simulink model "JXvoice"  (Simulink 7.7)
settings: Solver=ode45  StartTime=0.0  StopTime=10.0  RelTol=1e-3
undefined symbols (not defined in the file or in its folder): Fs, get, sided, Two
libraries: simulink x12, dspsrcs4 x2, dspmathops x1, dsparch4 x1, dspstat3 x1, dspsnks4 x1, dspsigops x1
settings Model: Creator=Jx  LastModifiedBy=Jx

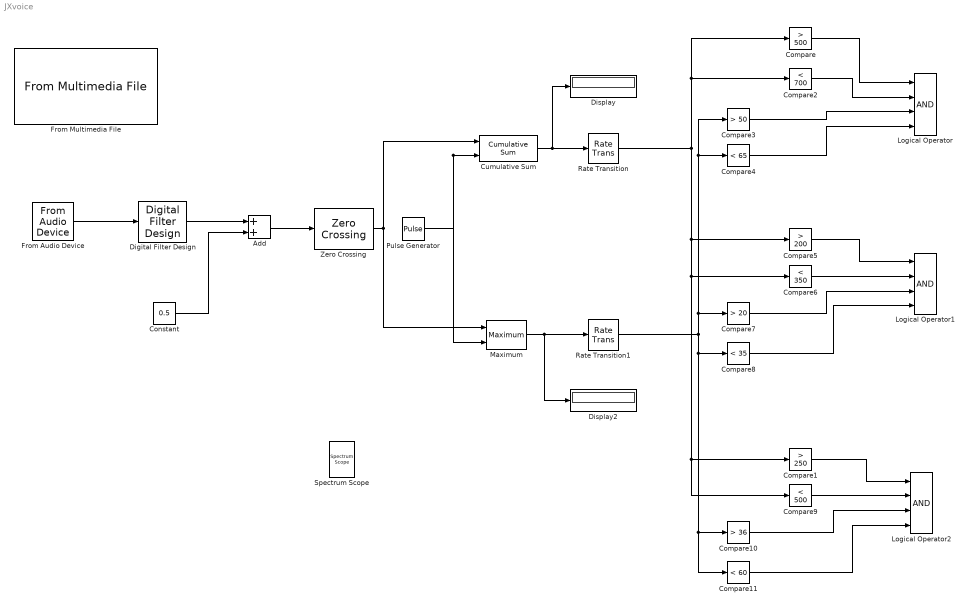
== system JXvoice ==
  Add : Sum
  Compare : simulink/Logic and Bit Operations/Compare To Constant  SystemSampleTime=-1  relop=>  const=500  LogicOutDataTypeMode=uint8
  Compare1 : simulink/Logic and Bit Operations/Compare To Constant  SystemSampleTime=-1  relop=>  const=250  LogicOutDataTypeMode=uint8
  Compare10 : simulink/Logic and Bit Operations/Compare To Constant  SystemSampleTime=-1  relop=>  const=36  LogicOutDataTypeMode=uint8
  Compare11 : simulink/Logic and Bit Operations/Compare To Constant  SystemSampleTime=-1  relop=<  const=60  LogicOutDataTypeMode=uint8
  Compare2 : simulink/Logic and Bit Operations/Compare To Constant  SystemSampleTime=-1  relop=<  const=700  LogicOutDataTypeMode=uint8
  Compare3 : simulink/Logic and Bit Operations/Compare To Constant  SystemSampleTime=-1  relop=>  const=50  LogicOutDataTypeMode=uint8
  Compare4 : simulink/Logic and Bit Operations/Compare To Constant  SystemSampleTime=-1  relop=<  const=65  LogicOutDataTypeMode=uint8
  Compare5 : simulink/Logic and Bit Operations/Compare To Constant  SystemSampleTime=-1  relop=>  const=200  LogicOutDataTypeMode=uint8
  Compare6 : simulink/Logic and Bit Operations/Compare To Constant  SystemSampleTime=-1  relop=<  const=350  LogicOutDataTypeMode=uint8
  Compare7 : simulink/Logic and Bit Operations/Compare To Constant  SystemSampleTime=-1  relop=>  const=20  LogicOutDataTypeMode=uint8
  Compare8 : simulink/Logic and Bit Operations/Compare To Constant  SystemSampleTime=-1  relop=<  const=35  LogicOutDataTypeMode=uint8
  Compare9 : simulink/Logic and Bit Operations/Compare To Constant  SystemSampleTime=-1  relop=<  const=500  LogicOutDataTypeMode=uint8
  Constant : Constant  Value=0.5
  Cumulative Sum : dspmathops/Cumulative Sum  dim=Channels (running sum)  InputProcessing=Columns as channels (frame based)  reset_popup=Either edge  outputDataTypeStr=Inherit: Same as accumulator  outputLastDataTypeStr=Inherit: Same as accumulator  outputMin=[]  outputMax=[]  roundingMode=Floor  overflowMode=off
  Digital Filter Design : dsparch4/Digital Filter Design  SystemSampleTime=-1  mwdsp_browser_bugfix_var=off
  Display : Display
  Display2 : Display
  From Audio Device : dspsrcs4/From Audio Device  deviceName=Default  numChannels=1  sampleRate=8000  deviceDatatype=24-bit integer  autoBufferSize=on  bufferSize=4096  queueDuration=1.0  frameSize=256  outputDatatype=single
  From Multimedia File : dspsrcs4/From Multimedia File  inputFilename=speech_dft.avi  loop=on  numPlays=inf  outputStreams=Audio only  videoDataType=single  audioDataType=int16  inheritSampleTime=on  userDefinedSampleTime=1/31.25  noAudioOutput=off  isIntensityVideo=off  fourcc=RGB  colorVideoFormat=Separate color signals  outputEOF=off  dataOrg=Column-major  audioFrameSize=5632  computeAudioFrameSize=off
  Logical Operator : Logic  Inputs=4  AllPortsSameDT=off  OutDataTypeStr=boolean
  Logical Operator1 : Logic  Inputs=4  AllPortsSameDT=off  OutDataTypeStr=boolean
  Logical Operator2 : Logic  Inputs=4  AllPortsSameDT=off  OutDataTypeStr=boolean
  Maximum : dspstat3/Maximum  fcn=Running  reset=Either edge  InputProcessing=Columns as channels (frame based)  indexBase=One  operateOver=Each column  Dimension=1  colComp=on  operation=maximum  roiEnable=off  roiType=Rectangles  roiPortion=Entire ROI  roiOutput=Individual statistics for each ROI  roiFlag=off  accumDataTypeStr=Inherit: Same as product output  accumLastDataTypeStr=Inherit: Same as product output  roundingMode=Floor  overflowMode=off
  Pulse Generator : DiscretePulseGenerator  SampleTime=1/31.25
  Rate Transition : RateTransition
  Rate Transition1 : RateTransition
  Spectrum Scope : dspsnks4/Spectrum Scope  SystemSampleTime=-1  ScopeProperties=on  Domain=Frequency  HorizSpan=1  UseBuffer=off  BufferSize=128  Overlap=0  TreatMby1Signals=One channel  inpFftLenInherit=off  FFTlength=128  numAvg=2  DisplayProperties=off  AxisGrid=on  Memory=off  FrameNumber=on  AxisLegend=off  AxisZoom=off  OpenScopeAtSimStart=on  OpenScopeImmediately=off  FigPos=get(0,'defaultfigureposition')  AxisProperties=off  XUnits=Hertz  XRange=Two-sided ((-Fs/2...Fs/2])  XDisplay=0  InheritXIncr=on  XIncr=1.0  XLabel=Samples  XLimit=Auto  YUnits=dBW/Hertz  XMax=1  XMin=0  YLabel=Magnitude-squared, dB  LineProperties=off  wintypeSpecScope=Hann  RsSpecScope=50  betaSpecScope=5  winsampSpecScope=Periodic  XAxisParamsVer=6.9  isFrameUpgraded=on
      settings: YMin=-10  YMax=10
  Zero Crossing : dspsigops/Zero Crossing  InputProcessing=Columns as channels (frame based)
  wires:
  Digital Filter Design/1 -> Add/1
  Constant/1 -> Add/2
  Add/1 -> Zero Crossing/1
  Zero Crossing/1 -> Maximum/1, Cumulative Sum/1
  Pulse Generator/1 -> Maximum/2, Cumulative Sum/2
  Cumulative Sum/1 -> Rate Transition/1, Display/1
  Maximum/1 -> Rate Transition1/1, Display2/1
  Rate Transition1/1 -> Compare3/1, Compare4/1, Compare7/1, Compare8/1, Compare10/1, Compare11/1
  Rate Transition/1 -> Compare/1, Compare2/1, Compare5/1, Compare6/1, Compare1/1, Compare9/1
  Compare/1 -> Logical Operator/1
  Compare2/1 -> Logical Operator/2
  Compare3/1 -> Logical Operator/3
  Compare4/1 -> Logical Operator/4
  Compare5/1 -> Logical Operator1/1
  Compare6/1 -> Logical Operator1/2
  Compare7/1 -> Logical Operator1/3
  Compare8/1 -> Logical Operator1/4
  Compare1/1 -> Logical Operator2/1
  Compare9/1 -> Logical Operator2/2
  Compare10/1 -> Logical Operator2/3
  Compare11/1 -> Logical Operator2/4
  From Audio Device/1 -> Digital Filter Design/1
